simulink model "Modelesimulink_l2p1"  (Simulink 8.7)
settings: Solver=ode3  StartTime=0.0  StopTime=0.001  FixedStep=0.0001  RelTol=1e-3
values from neighbouring files (symbols this model uses):
  C = [2*cA1+cA2 -cA2 -2*cA1 -2*Lar*cA1+Lav*cA2;-cA2 cA2 0 -Lav*cA2;-2*cA1 0 2*cA1 2*Lar*cA1; -2*Lar*cA1+Lav*cA2 -Lav*cA2 2*Lar*cA1 2*Lar^2*cA1+Lav^2*cA2]    [labo2p1.m]
  F = [0;kN*f;2*kM*f;0]    [labo2p1.m]
  K = [(2*kA1+kA2) -kA2 -2*kA1 -2*kA1*Lar+kA2*Lav; -kA2 kA2+kN 0 -Lav*kA2; -2*kA1 0 2*(kA1+kM) 2*kA1*Lar; -2*kA1*Lar+kA2*Lav -Lav*kA2 2*kA1*Lar Lav^2*kA2+2*Lar^2*kA1]    [labo2p1.m]
  M = [Ma 0 0 0;0 Mn 0 0;0 0 M2m 0;0 0 0 I]    [labo2p1.m]
  Phi = [0;0;-2.77;0]    [labo2p1.m]
undefined symbols (not defined in the file or in its folder): w
settings Model: Creator=p202400  LastModifiedBy=User
settings DataIOCC: SignalLoggingSaveFormat=ModelDataLogs
settings OptimizationCC: ExpressionDepthLimit=2147483647
settings DebuggingCC: SolverPrmCheckMsg=warning  FcnCallInpInsideContextMsg=UseLocalSettings  StateNameClashWarn=warning
settings GRTTargetCC: CombineOutputUpdateFcns=off  GRTInterface=on

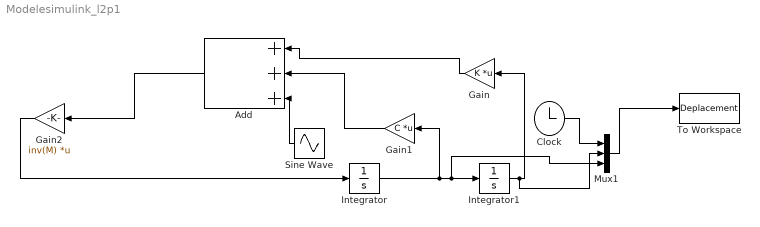
== system Modelesimulink_l2p1 ==
  Add : Sum  Inputs=+++
  Clock : Clock
  Gain : Gain  Gain=K  Multiplication=Matrix(K*u) (u vector)
  Gain1 : Gain  Gain=C  Multiplication=Matrix(K*u) (u vector)
  Gain2 : Gain  Gain=inv(M)  Multiplication=Matrix(K*u) (u vector)
  Integrator : Integrator
  Integrator1 : Integrator
  Mux1 : Mux  Inputs=3
  Sine Wave : Sin  Amplitude=F  Frequency=w  Phase=Phi  SampleTime=0
  To Workspace : ToWorkspace  VariableName=Deplacement  SampleTime=-1
  wires:
  Integrator/1 -> Mux1/3, Integrator1/1, Gain1/1
  Integrator1/1 -> Gain/1, Mux1/2
  Gain1/1 -> Add/2
  Gain/1 -> Add/1
  Clock/1 -> Mux1/1
  Mux1/1 -> To Workspace/1
  Sine Wave/1 -> Add/3
  Gain2/1 -> Integrator/1
  Add/1 -> Gain2/1
